simulink model "TSR_Scenario_001_cs"  (R2014b)
settings: Solver=ode5  SolverMode=SingleTasking  StartTime=0.0  StopTime=inf  FixedStep=1/100  RelTol=1e-3
PreLoadFcn:
  | mbxruntime.callbacks.PreLoadFcn(bdroot);
  | check_NUTS_defined;
  | 
  | assignin('base',['model_closed_' bdroot],false);
  | 
  | addpath('../includes_TSR/includes_TSR');
  | 
  | switch version('-release')
  | case {'2010a', '2010b', '2011a'}
  | addpath('../includes_TSR/ML2010b');
  | otherwise
  | addpath('../includes_TSR/ML2011b');
  | end
PostLoadFcn:
  | mbxruntime.callbacks.PostLoadFcn(bdroot);
InitFcn:
  | mbxruntime.callbacks.InitFcn(bdroot);
StartFcn:
  | mbxruntime.callbacks.StartFcn(bdroot);
StopFcn:
  | mbxruntime.callbacks.StopFcn(bdroot);
model workspace: external: MAT-File .\TSR_Scenario_001_cs_hws.mat (data not in the file)
undefined symbols (not defined in the file or in its folder): InitImageOutputDir, mbxruntime, OrientationPitch, OrientationRoll, PositionX, PositionY, PositionZ, tabledata, warningInitialVelocity, x0
undefined symbols (not defined in the file): SteeringColumn, SteeringWheel, TSR_Scenario_001_cs_0469e6db089af631, TSR_Scenario_001_cs_0511100212e7bc8e, TSR_Scenario_001_cs_0e7e9ae969427aac, TSR_Scenario_001_cs_1093386e49c2fe1f, TSR_Scenario_001_cs_112063adae8cf595, TSR_Scenario_001_cs_20f00d93cd5331c2, TSR_Scenario_001_cs_23e3512474fbfadc, TSR_Scenario_001_cs_366523e1554c6bf4, TSR_Scenario_001_cs_37bce4982c67337a, TSR_Scenario_001_cs_44e6164a5df50f45, TSR_Scenario_001_cs_4963ce12e7ff3247, TSR_Scenario_001_cs_4b3e01fa729ce73a, TSR_Scenario_001_cs_519c34727ce9f069, TSR_Scenario_001_cs_5b66ab60038399a1, TSR_Scenario_001_cs_5baa165dfa1afdcb, TSR_Scenario_001_cs_5f993ce39fa6372c, TSR_Scenario_001_cs_613fdf28e3ff7437, TSR_Scenario_001_cs_67b1406af835d622, TSR_Scenario_001_cs_6ad990c290286b94, TSR_Scenario_001_cs_6c412b69295984e1, TSR_Scenario_001_cs_6d4c0c06b1585ef3, TSR_Scenario_001_cs_6dd019d071bf1235, TSR_Scenario_001_cs_6e9f5883f1a78533, TSR_Scenario_001_cs_80f7223d9ac35404, TSR_Scenario_001_cs_8562b82d3c89ae57, TSR_Scenario_001_cs_8a3a0181ab0babfe, TSR_Scenario_001_cs_8c997348ce80deaf, TSR_Scenario_001_cs_925bd6a073d9fe25, TSR_Scenario_001_cs_961436216add6114, TSR_Scenario_001_cs_991a7959256b2c84, TSR_Scenario_001_cs_9a95ce2c2e753616, TSR_Scenario_001_cs_a98aa9562e8552a9, TSR_Scenario_001_cs_ab44ae81dbfb58cd, TSR_Scenario_001_cs_Actros_2541_2_Path_pathUniqueID, TSR_Scenario_001_cs_ae74836ade6bff5a, TSR_Scenario_001_cs_Audi_A8_1_Dynamics_Simple_initialPitch, TSR_Scenario_001_cs_Audi_A8_1_Dynamics_Simple_initialRoll, TSR_Scenario_001_cs_Audi_A8_1_Dynamics_Simple_initialX, TSR_Scenario_001_cs_Audi_A8_1_Dynamics_Simple_initialY, TSR_Scenario_001_cs_Audi_A8_1_Dynamics_Simple_initialYaw, TSR_Scenario_001_cs_Audi_A8_1_Dynamics_Simple_initialZ, TSR_Scenario_001_cs_Audi_A8_2_Path_pathUniqueID, TSR_Scenario_001_cs_Audi_A8_2_SpeedProfile_speedProfileUniqueID, TSR_Scenario_001_cs_b2eca4eb2fce349a, TSR_Scenario_001_cs_b7bac209c1f2549f, TSR_Scenario_001_cs_bf3dccb66d3255a4, TSR_Scenario_001_cs_bf4c1a5315e3f716, TSR_Scenario_001_cs_BMW_Z3_1_Path_pathUniqueID, TSR_Scenario_001_cs_BMW_Z3_1_SpeedProfile_speedProfileUniqueID, TSR_Scenario_001_cs_BMW_Z3_2_Path_pathUniqueID, TSR_Scenario_001_cs_BMW_Z3_2_SpeedProfile_speedProfileUniqueID, TSR_Scenario_001_cs_c4c8fc4bdece03a9, TSR_Scenario_001_cs_c964c86aa54ad92e, TSR_Scenario_001_cs_cb64d1ef85329755, TSR_Scenario_001_cs_Citroen_C3_1_Path_pathUniqueID, TSR_Scenario_001_cs_Citroen_C3_2_Path_pathUniqueID, TSR_Scenario_001_cs_Citroen_C3_3_Path_pathUniqueID, TSR_Scenario_001_cs_Citroen_C3_4_Path_pathUniqueID ... (+25)
libraries: simulink x21, PreScanSimulinkLibrary x17, simulink_extras x13
(part 7 of 30)

== system TSR_Scenario_001_cs/Toyota_Yaris_1 ==
  SELF_Toyota_Yaris_1 : Inport  Tag=inport/SelfPort  OutDataTypeStr=Bus: PRESCAN_SELFSENSORDATA  PortDimensions=1  SampleTime=1/100  BusOutputAsStruct=on
  ColorRegion_Exterior_color : Constant  Tag=VisuLightConst  Value=[255 255 224]
  Ground_{1..6} (6 alike) : Ground
  JointGroup_WheelDisplacement_V2R : Subsystem  Tag=mux/Wheels  mask(PreScan Velocity to Wheel Angle Block:){TimeStep=1/100, TireRadius=0.29}
      mask prompts: TimeStep "Auto Assigned: Time Step [s]"; TireRadius "Tire Radius [m]"
      settings: DeleteFcn=PreScanBlockDeleteFcn;
      mask Display: disp('Velocity\nto\nWheelAngle')
  Path : S-Function  Tag=Path  LoadFcn=load('PrescanMotionData.mat')  FunctionName=sfun_Path  Parameters=uniqueID, pathUniqueID, timestep  EnableBusSupport=off  mask(Path){uniqueID=1961, pathUniqueID=TSR_Scenario_001_cs_Toyota_Yaris_1_Path_pathUniqueID, timestep=1/100}
      mask prompts: uniqueID "Object Unique ID"; pathUniqueID "Path Unique ID"; timestep "MATLAB timestep:"
      mask help:
      | The path block outputs the position along a given trajectory.
      |
      | For more information, please click Help.
      mask Help: eval('openHelp(312)')
      mask Display: image(imread('Path.png'))
  SELF_Demux : Subsystem  Tag=demux/SelfPort  mask(PreScan Demux Block:){}
      mask help:
      | The SELF port shows (state) information of the actor itself. The outputs are position in the experiment's axis system and the GPS coordinates, and the object's absolute velocity and compass heading.
      |
      | For more information, please click Help.
      settings: DeleteFcn=PreScanBlockDeleteFcn;
      mask Help: eval('openHelp(462)')
      mask Display:
      | port_label('output',1,'x [m]')
      | port_label('output',2,'y [m]')
      | port_label('output',3,'z [m]','texmode','on')
      | port_label('output',4,'Rotx [deg]','texmode','on')
      | port_label('output',5,'Roty [deg]','texmode','on')
      | port_label('output',6,'Rotz [deg]','texmode','on')
      | port_label('output',7,'GPS lat [deg]','texmode','on')
      | port_label('output',8,'GPS long [deg]','texmode','on')
      | port_label('output',9,'GPS alt [m]','texmode','on')
      | port_label('output',10,'Velocity [m/s]')
      | port_label('output',11,'Heading [deg]')
      | port_label('output',12,'Yaw rate [deg/s]')
  STATE_Toyota_Yaris_1_rc : RateTransition  Tag=mux_rc/StatePort  OutPortSampleTimeOpt=Inherit
  SpeedProfile : S-Function  Tag=SpeedProfile  LoadFcn=load('PrescanMotionData.mat')  FunctionName=sfun_SpeedProfile  Parameters=speedProfileUniqueID, timestep  EnableBusSupport=off  mask(SpeedProfile){speedProfileUniqueID=TSR_Scenario_001_cs_dadaf9392218b438, timestep=1/100}
      mask prompts: speedProfileUniqueID "Speed Profile Unique ID"; timestep "MATLAB timestep:"
      mask help:
      | The speed profile block outputs the travelled distance, velocities and acceleration along a given path.
      |
      | For more information, please click Help.
      mask Help: eval('openHelp(312)')
      mask Display: image(imread('SpeedProfile.png'))
  Terminator_{1..11} (11 alike) : Terminator
  VISUColorRegion_Exterior_Mux : Subsystem  Tag=mux/MuxColorRegion  LoadFcn=load PrescanColorData  mask(PreScan User Interface: VisuTextureColor){}
      mask help:
      | The VisuTextureColor block provides a way to adapt the color of a vehicle.
      |
      | For more information, please click Help.
      settings: DeleteFcn=PreScanBlockDeleteFcn;
      mask Help: eval('openHelp(230)')
  WheelDisplacement_Mux : Subsystem  Tag=mux/JointGroup  mask(JointGroup){}
      mask help:
      | The JointGroup allows to control several Joints in one go, as defined for this particular model.
      | For more information, look in the PreScan manual in the section "Model Preparation Tool" -> "Joint Groups"
      |
      | For more information on the Joints simulink interface, press Help.
      mask Help: eval('openHelp(254)')
  STATE_Toyota_Yaris_1_bus : Outport  Tag=outport/StatePort  OutDataTypeStr=Bus: PRESCAN_STATEACTUATORDATA  PortDimensions=1  SampleTime=1/100
  WheelL0_Toyota_Yaris_1 : Outport  Tag=outport/JointActuator  Port=2  OutDataTypeStr=Bus: PRESCAN_POSE_DATA  SampleTime=1/100
  WheelL1_Toyota_Yaris_1 : Outport  Tag=outport/JointActuator  Port=3  OutDataTypeStr=Bus: PRESCAN_POSE_DATA  SampleTime=1/100
  WheelR0_Toyota_Yaris_1 : Outport  Tag=outport/JointActuator  Port=4  OutDataTypeStr=Bus: PRESCAN_POSE_DATA  SampleTime=1/100
  WheelR1_Toyota_Yaris_1 : Outport  Tag=outport/JointActuator  Port=5  OutDataTypeStr=Bus: PRESCAN_POSE_DATA  SampleTime=1/100
  VISUColorRegion_Exterior_Toyota_Yaris_1 : Outport  Tag=outport/ColorRegion  Port=6  OutDataTypeStr=Bus: PRESCAN_COLOR_DATA  PortDimensions=1  SampleTime=1/100
  wires:
  SELF_Demux/10(velocity [m/s]) -> JointGroup_WheelDisplacement_V2R/1(Velocity [m/s])
  STATE_Toyota_Yaris_1_rc/1 -> STATE_Toyota_Yaris_1_bus/1
  SpeedProfile/1 -> Path/1
  Path/1 -> STATE_Toyota_Yaris_1_rc/1
  SELF_Toyota_Yaris_1/1 -> SELF_Demux/1(SELF)
  WheelDisplacement_Mux/1(WheelL0_Toyota_Yaris_1) -> WheelL0_Toyota_Yaris_1/1
  WheelDisplacement_Mux/2(WheelL1_Toyota_Yaris_1) -> WheelL1_Toyota_Yaris_1/1
  WheelDisplacement_Mux/3(WheelR0_Toyota_Yaris_1) -> WheelR0_Toyota_Yaris_1/1
  WheelDisplacement_Mux/4(WheelR1_Toyota_Yaris_1) -> WheelR1_Toyota_Yaris_1/1
  JointGroup_WheelDisplacement_V2R/1(Rotation [rad]) -> WheelDisplacement_Mux/3(Rotation [rad])
  VISUColorRegion_Exterior_Mux/1(ColorRegion) -> VISUColorRegion_Exterior_Toyota_Yaris_1/1
  ColorRegion_Exterior_color/1 -> VISUColorRegion_Exterior_Mux/1(RGB [-,-,-])
  SELF_Demux/1(x [m]) -> Terminator_1/1
  SELF_Demux/2(y [m]) -> Terminator_2/1
  SELF_Demux/3(z [m]) -> Terminator_3/1
  SELF_Demux/4(rotx [deg]) -> Terminator_4/1
  SELF_Demux/5(roty [deg]) -> Terminator_5/1
  SELF_Demux/6(rotz [deg]) -> Terminator_6/1
  SELF_Demux/7(GPS lat [deg]) -> Terminator_7/1
  SELF_Demux/8(GPS long [deg]) -> Terminator_8/1
  SELF_Demux/9(GPS alt [m]) -> Terminator_9/1
  SELF_Demux/11(heading [deg]) -> Terminator_10/1
  SELF_Demux/12(yaw rate [deg/s]) -> Terminator_11/1
  Ground_1/1 -> WheelDisplacement_Mux/1(Steering Angle Front [rad])
  Ground_2/1 -> WheelDisplacement_Mux/2(Steering Angle Rear [rad])
  Ground_3/1 -> WheelDisplacement_Mux/4(zDisp FL [m])
  Ground_4/1 -> WheelDisplacement_Mux/5(zDisp FR [m])
  Ground_5/1 -> WheelDisplacement_Mux/6(zDisp RL [m])
  Ground_6/1 -> WheelDisplacement_Mux/7(zDisp RR [m])

== system TSR_Scenario_001_cs/VISUColorRegion_Exterior_Audi_A8_2 ==
  VISUColorRegion_Exterior_Audi_A8_2 : Inport  Tag=inport/ColorRegion  OutDataTypeStr=Bus: PRESCAN_COLOR_DATA  PortDimensions=1  SampleTime=1/100  BusOutputAsStruct=on
  Actuator : S-Function  FunctionName=sfun_ColorActuator  Parameters=mbxruntime.parameters.convert(UniqueID), mbxruntime.parameters.convert(WorldModelSubPath),tabledata, TimeStep  EnableBusSupport=off  mask(PreScan Sink Block: VisuTextureColor){UniqueID=1951, WorldModelSubPath=/recolorRegion:name=Exterior/targetColor, TimeStep=1/100}
      mask prompts: UniqueID "Parent Unique Identifier (auto-generated)"; WorldModelSubPath "WM SubPath(auto-generated)"; TimeStep "Simulink time step"
      mask help:
      | The VisuTextureColor block provides a way to adapt the color of a vehicle.
      |
      | For more information, please click Help.
      mask init:
      | [tabledata] = mbxruntime.parameters.table(UniqueID,WorldModelSubPath);
      mask Help: eval('openHelp(230)')
      mask Display: image(imread('TextureColor.png'))
  wires:
  VISUColorRegion_Exterior_Audi_A8_2/1 -> Actuator/1

== system TSR_Scenario_001_cs/VISUColorRegion_Exterior_BMW_Z3_1 ==
  VISUColorRegion_Exterior_BMW_Z3_1 : Inport  Tag=inport/ColorRegion  OutDataTypeStr=Bus: PRESCAN_COLOR_DATA  PortDimensions=1  SampleTime=1/100  BusOutputAsStruct=on
  Actuator : S-Function  FunctionName=sfun_ColorActuator  Parameters=mbxruntime.parameters.convert(UniqueID), mbxruntime.parameters.convert(WorldModelSubPath),tabledata, TimeStep  EnableBusSupport=off  mask(PreScan Sink Block: VisuTextureColor){UniqueID=1948, WorldModelSubPath=/recolorRegion:name=Exterior/targetColor, TimeStep=1/100}
      mask prompts: UniqueID "Parent Unique Identifier (auto-generated)"; WorldModelSubPath "WM SubPath(auto-generated)"; TimeStep "Simulink time step"
      mask help:
      | The VisuTextureColor block provides a way to adapt the color of a vehicle.
      |
      | For more information, please click Help.
      mask init:
      | [tabledata] = mbxruntime.parameters.table(UniqueID,WorldModelSubPath);
      mask Help: eval('openHelp(230)')
      mask Display: image(imread('TextureColor.png'))
  wires:
  VISUColorRegion_Exterior_BMW_Z3_1/1 -> Actuator/1

== system TSR_Scenario_001_cs/VISUColorRegion_Exterior_BMW_Z3_2 ==
  VISUColorRegion_Exterior_BMW_Z3_2 : Inport  Tag=inport/ColorRegion  OutDataTypeStr=Bus: PRESCAN_COLOR_DATA  PortDimensions=1  SampleTime=1/100  BusOutputAsStruct=on
  Actuator : S-Function  FunctionName=sfun_ColorActuator  Parameters=mbxruntime.parameters.convert(UniqueID), mbxruntime.parameters.convert(WorldModelSubPath),tabledata, TimeStep  EnableBusSupport=off  mask(PreScan Sink Block: VisuTextureColor){UniqueID=2024, WorldModelSubPath=/recolorRegion:name=Exterior/targetColor, TimeStep=1/100}
      mask prompts: UniqueID "Parent Unique Identifier (auto-generated)"; WorldModelSubPath "WM SubPath(auto-generated)"; TimeStep "Simulink time step"
      mask help:
      | The VisuTextureColor block provides a way to adapt the color of a vehicle.
      |
      | For more information, please click Help.
      mask init:
      | [tabledata] = mbxruntime.parameters.table(UniqueID,WorldModelSubPath);
      mask Help: eval('openHelp(230)')
      mask Display: image(imread('TextureColor.png'))
  wires:
  VISUColorRegion_Exterior_BMW_Z3_2/1 -> Actuator/1

== system TSR_Scenario_001_cs/VISUColorRegion_Exterior_Citroen_C3_1 ==
  VISUColorRegion_Exterior_Citroen_C3_1 : Inport  Tag=inport/ColorRegion  OutDataTypeStr=Bus: PRESCAN_COLOR_DATA  PortDimensions=1  SampleTime=1/100  BusOutputAsStruct=on
  Actuator : S-Function  FunctionName=sfun_ColorActuator  Parameters=mbxruntime.parameters.convert(UniqueID), mbxruntime.parameters.convert(WorldModelSubPath),tabledata, TimeStep  EnableBusSupport=off  mask(PreScan Sink Block: VisuTextureColor){UniqueID=1955, WorldModelSubPath=/recolorRegion:name=Exterior/targetColor, TimeStep=1/100}
      mask prompts: UniqueID "Parent Unique Identifier (auto-generated)"; WorldModelSubPath "WM SubPath(auto-generated)"; TimeStep "Simulink time step"
      mask help:
      | The VisuTextureColor block provides a way to adapt the color of a vehicle.
      |
      | For more information, please click Help.
      mask init:
      | [tabledata] = mbxruntime.parameters.table(UniqueID,WorldModelSubPath);
      mask Help: eval('openHelp(230)')
      mask Display: image(imread('TextureColor.png'))
  wires:
  VISUColorRegion_Exterior_Citroen_C3_1/1 -> Actuator/1

== system TSR_Scenario_001_cs/VISUColorRegion_Exterior_Citroen_C3_2 ==
  VISUColorRegion_Exterior_Citroen_C3_2 : Inport  Tag=inport/ColorRegion  OutDataTypeStr=Bus: PRESCAN_COLOR_DATA  PortDimensions=1  SampleTime=1/100  BusOutputAsStruct=on
  Actuator : S-Function  FunctionName=sfun_ColorActuator  Parameters=mbxruntime.parameters.convert(UniqueID), mbxruntime.parameters.convert(WorldModelSubPath),tabledata, TimeStep  EnableBusSupport=off  mask(PreScan Sink Block: VisuTextureColor){UniqueID=1958, WorldModelSubPath=/recolorRegion:name=Exterior/targetColor, TimeStep=1/100}
      mask prompts: UniqueID "Parent Unique Identifier (auto-generated)"; WorldModelSubPath "WM SubPath(auto-generated)"; TimeStep "Simulink time step"
      mask help:
      | The VisuTextureColor block provides a way to adapt the color of a vehicle.
      |
      | For more information, please click Help.
      mask init:
      | [tabledata] = mbxruntime.parameters.table(UniqueID,WorldModelSubPath);
      mask Help: eval('openHelp(230)')
      mask Display: image(imread('TextureColor.png'))
  wires:
  VISUColorRegion_Exterior_Citroen_C3_2/1 -> Actuator/1

== system TSR_Scenario_001_cs/VISUColorRegion_Exterior_Citroen_C3_3 ==
  VISUColorRegion_Exterior_Citroen_C3_3 : Inport  Tag=inport/ColorRegion  OutDataTypeStr=Bus: PRESCAN_COLOR_DATA  PortDimensions=1  SampleTime=1/100  BusOutputAsStruct=on
  Actuator : S-Function  FunctionName=sfun_ColorActuator  Parameters=mbxruntime.parameters.convert(UniqueID), mbxruntime.parameters.convert(WorldModelSubPath),tabledata, TimeStep  EnableBusSupport=off  mask(PreScan Sink Block: VisuTextureColor){UniqueID=1967, WorldModelSubPath=/recolorRegion:name=Exterior/targetColor, TimeStep=1/100}
      mask prompts: UniqueID "Parent Unique Identifier (auto-generated)"; WorldModelSubPath "WM SubPath(auto-generated)"; TimeStep "Simulink time step"
      mask help:
      | The VisuTextureColor block provides a way to adapt the color of a vehicle.
      |
      | For more information, please click Help.
      mask init:
      | [tabledata] = mbxruntime.parameters.table(UniqueID,WorldModelSubPath);
      mask Help: eval('openHelp(230)')
      mask Display: image(imread('TextureColor.png'))
  wires:
  VISUColorRegion_Exterior_Citroen_C3_3/1 -> Actuator/1

== system TSR_Scenario_001_cs/VISUColorRegion_Exterior_Citroen_C3_4 ==
  VISUColorRegion_Exterior_Citroen_C3_4 : Inport  Tag=inport/ColorRegion  OutDataTypeStr=Bus: PRESCAN_COLOR_DATA  PortDimensions=1  SampleTime=1/100  BusOutputAsStruct=on
  Actuator : S-Function  FunctionName=sfun_ColorActuator  Parameters=mbxruntime.parameters.convert(UniqueID), mbxruntime.parameters.convert(WorldModelSubPath),tabledata, TimeStep  EnableBusSupport=off  mask(PreScan Sink Block: VisuTextureColor){UniqueID=2027, WorldModelSubPath=/recolorRegion:name=Exterior/targetColor, TimeStep=1/100}
      mask prompts: UniqueID "Parent Unique Identifier (auto-generated)"; WorldModelSubPath "WM SubPath(auto-generated)"; TimeStep "Simulink time step"
      mask help:
      | The VisuTextureColor block provides a way to adapt the color of a vehicle.
      |
      | For more information, please click Help.
      mask init:
      | [tabledata] = mbxruntime.parameters.table(UniqueID,WorldModelSubPath);
      mask Help: eval('openHelp(230)')
      mask Display: image(imread('TextureColor.png'))
  wires:
  VISUColorRegion_Exterior_Citroen_C3_4/1 -> Actuator/1

== system TSR_Scenario_001_cs/VISUColorRegion_Exterior_Fiat_Bravo_1 ==
  VISUColorRegion_Exterior_Fiat_Bravo_1 : Inport  Tag=inport/ColorRegion  OutDataTypeStr=Bus: PRESCAN_COLOR_DATA  PortDimensions=1  SampleTime=1/100  BusOutputAsStruct=on
  Actuator : S-Function  FunctionName=sfun_ColorActuator  Parameters=mbxruntime.parameters.convert(UniqueID), mbxruntime.parameters.convert(WorldModelSubPath),tabledata, TimeStep  EnableBusSupport=off  mask(PreScan Sink Block: VisuTextureColor){UniqueID=1964, WorldModelSubPath=/recolorRegion:name=Exterior/targetColor, TimeStep=1/100}
      mask prompts: UniqueID "Parent Unique Identifier (auto-generated)"; WorldModelSubPath "WM SubPath(auto-generated)"; TimeStep "Simulink time step"
      mask help:
      | The VisuTextureColor block provides a way to adapt the color of a vehicle.
      |
      | For more information, please click Help.
      mask init:
      | [tabledata] = mbxruntime.parameters.table(UniqueID,WorldModelSubPath);
      mask Help: eval('openHelp(230)')
      mask Display: image(imread('TextureColor.png'))
  wires:
  VISUColorRegion_Exterior_Fiat_Bravo_1/1 -> Actuator/1

== system TSR_Scenario_001_cs/VISUColorRegion_Exterior_Ford_Fiesta_1 ==
  VISUColorRegion_Exterior_Ford_Fiesta_1 : Inport  Tag=inport/ColorRegion  OutDataTypeStr=Bus: PRESCAN_COLOR_DATA  PortDimensions=1  SampleTime=1/100  BusOutputAsStruct=on
  Actuator : S-Function  FunctionName=sfun_ColorActuator  Parameters=mbxruntime.parameters.convert(UniqueID), mbxruntime.parameters.convert(WorldModelSubPath),tabledata, TimeStep  EnableBusSupport=off  mask(PreScan Sink Block: VisuTextureColor){UniqueID=1934, WorldModelSubPath=/recolorRegion:name=Exterior/targetColor, TimeStep=1/100}
      mask prompts: UniqueID "Parent Unique Identifier (auto-generated)"; WorldModelSubPath "WM SubPath(auto-generated)"; TimeStep "Simulink time step"
      mask help:
      | The VisuTextureColor block provides a way to adapt the color of a vehicle.
      |
      | For more information, please click Help.
      mask init:
      | [tabledata] = mbxruntime.parameters.table(UniqueID,WorldModelSubPath);
      mask Help: eval('openHelp(230)')
      mask Display: image(imread('TextureColor.png'))
  wires:
  VISUColorRegion_Exterior_Ford_Fiesta_1/1 -> Actuator/1

== system TSR_Scenario_001_cs/VISUColorRegion_Exterior_Mazda_RX8_1 ==
  VISUColorRegion_Exterior_Mazda_RX8_1 : Inport  Tag=inport/ColorRegion  OutDataTypeStr=Bus: PRESCAN_COLOR_DATA  PortDimensions=1  SampleTime=1/100  BusOutputAsStruct=on
  Actuator : S-Function  FunctionName=sfun_ColorActuator  Parameters=mbxruntime.parameters.convert(UniqueID), mbxruntime.parameters.convert(WorldModelSubPath),tabledata, TimeStep  EnableBusSupport=off  mask(PreScan Sink Block: VisuTextureColor){UniqueID=1863, WorldModelSubPath=/recolorRegion:name=Exterior/targetColor, TimeStep=1/100}
      mask prompts: UniqueID "Parent Unique Identifier (auto-generated)"; WorldModelSubPath "WM SubPath(auto-generated)"; TimeStep "Simulink time step"
      mask help:
      | The VisuTextureColor block provides a way to adapt the color of a vehicle.
      |
      | For more information, please click Help.
      mask init:
      | [tabledata] = mbxruntime.parameters.table(UniqueID,WorldModelSubPath);
      mask Help: eval('openHelp(230)')
      mask Display: image(imread('TextureColor.png'))
  wires:
  VISUColorRegion_Exterior_Mazda_RX8_1/1 -> Actuator/1

== system TSR_Scenario_001_cs/VISUColorRegion_Exterior_Mazda_RX8_2 ==
  VISUColorRegion_Exterior_Mazda_RX8_2 : Inport  Tag=inport/ColorRegion  OutDataTypeStr=Bus: PRESCAN_COLOR_DATA  PortDimensions=1  SampleTime=1/100  BusOutputAsStruct=on
  Actuator : S-Function  FunctionName=sfun_ColorActuator  Parameters=mbxruntime.parameters.convert(UniqueID), mbxruntime.parameters.convert(WorldModelSubPath),tabledata, TimeStep  EnableBusSupport=off  mask(PreScan Sink Block: VisuTextureColor){UniqueID=1929, WorldModelSubPath=/recolorRegion:name=Exterior/targetColor, TimeStep=1/100}
      mask prompts: UniqueID "Parent Unique Identifier (auto-generated)"; WorldModelSubPath "WM SubPath(auto-generated)"; TimeStep "Simulink time step"
      mask help:
      | The VisuTextureColor block provides a way to adapt the color of a vehicle.
      |
      | For more information, please click Help.
      mask init:
      | [tabledata] = mbxruntime.parameters.table(UniqueID,WorldModelSubPath);
      mask Help: eval('openHelp(230)')
      mask Display: image(imread('TextureColor.png'))
  wires:
  VISUColorRegion_Exterior_Mazda_RX8_2/1 -> Actuator/1

== system TSR_Scenario_001_cs/VISUColorRegion_Exterior_Mazda_RX8_3 ==
  VISUColorRegion_Exterior_Mazda_RX8_3 : Inport  Tag=inport/ColorRegion  OutDataTypeStr=Bus: PRESCAN_COLOR_DATA  PortDimensions=1  SampleTime=1/100  BusOutputAsStruct=on
  Actuator : S-Function  FunctionName=sfun_ColorActuator  Parameters=mbxruntime.parameters.convert(UniqueID), mbxruntime.parameters.convert(WorldModelSubPath),tabledata, TimeStep  EnableBusSupport=off  mask(PreScan Sink Block: VisuTextureColor){UniqueID=1973, WorldModelSubPath=/recolorRegion:name=Exterior/targetColor, TimeStep=1/100}
      mask prompts: UniqueID "Parent Unique Identifier (auto-generated)"; WorldModelSubPath "WM SubPath(auto-generated)"; TimeStep "Simulink time step"
      mask help:
      | The VisuTextureColor block provides a way to adapt the color of a vehicle.
      |
      | For more information, please click Help.
      mask init:
      | [tabledata] = mbxruntime.parameters.table(UniqueID,WorldModelSubPath);
      mask Help: eval('openHelp(230)')
      mask Display: image(imread('TextureColor.png'))
  wires:
  VISUColorRegion_Exterior_Mazda_RX8_3/1 -> Actuator/1

== system TSR_Scenario_001_cs/VISUColorRegion_Exterior_Nissan_Cabstar_1 ==
  VISUColorRegion_Exterior_Nissan_Cabstar_1 : Inport  Tag=inport/ColorRegion  OutDataTypeStr=Bus: PRESCAN_COLOR_DATA  PortDimensions=1  SampleTime=1/100  BusOutputAsStruct=on
  Actuator : S-Function  FunctionName=sfun_ColorActuator  Parameters=mbxruntime.parameters.convert(UniqueID), mbxruntime.parameters.convert(WorldModelSubPath),tabledata, TimeStep  EnableBusSupport=off  mask(PreScan Sink Block: VisuTextureColor){UniqueID=1579, WorldModelSubPath=/recolorRegion:name=Exterior/targetColor, TimeStep=1/100}
      mask prompts: UniqueID "Parent Unique Identifier (auto-generated)"; WorldModelSubPath "WM SubPath(auto-generated)"; TimeStep "Simulink time step"
      mask help:
      | The VisuTextureColor block provides a way to adapt the color of a vehicle.
      |
      | For more information, please click Help.
      mask init:
      | [tabledata] = mbxruntime.parameters.table(UniqueID,WorldModelSubPath);
      mask Help: eval('openHelp(230)')
      mask Display: image(imread('TextureColor.png'))
  wires:
  VISUColorRegion_Exterior_Nissan_Cabstar_1/1 -> Actuator/1

== system TSR_Scenario_001_cs/VISUColorRegion_Exterior_Toyota_Previa_1 ==
  VISUColorRegion_Exterior_Toyota_Previa_1 : Inport  Tag=inport/ColorRegion  OutDataTypeStr=Bus: PRESCAN_COLOR_DATA  PortDimensions=1  SampleTime=1/100  BusOutputAsStruct=on
  Actuator : S-Function  FunctionName=sfun_ColorActuator  Parameters=mbxruntime.parameters.convert(UniqueID), mbxruntime.parameters.convert(WorldModelSubPath),tabledata, TimeStep  EnableBusSupport=off  mask(PreScan Sink Block: VisuTextureColor){UniqueID=1688, WorldModelSubPath=/recolorRegion:name=Exterior/targetColor, TimeStep=1/100}
      mask prompts: UniqueID "Parent Unique Identifier (auto-generated)"; WorldModelSubPath "WM SubPath(auto-generated)"; TimeStep "Simulink time step"
      mask help:
      | The VisuTextureColor block provides a way to adapt the color of a vehicle.
      |
      | For more information, please click Help.
      mask init:
      | [tabledata] = mbxruntime.parameters.table(UniqueID,WorldModelSubPath);
      mask Help: eval('openHelp(230)')
      mask Display: image(imread('TextureColor.png'))
  wires:
  VISUColorRegion_Exterior_Toyota_Previa_1/1 -> Actuator/1

== system TSR_Scenario_001_cs/VISUColorRegion_Exterior_Toyota_Previa_2 ==
  VISUColorRegion_Exterior_Toyota_Previa_2 : Inport  Tag=inport/ColorRegion  OutDataTypeStr=Bus: PRESCAN_COLOR_DATA  PortDimensions=1  SampleTime=1/100  BusOutputAsStruct=on
  Actuator : S-Function  FunctionName=sfun_ColorActuator  Parameters=mbxruntime.parameters.convert(UniqueID), mbxruntime.parameters.convert(WorldModelSubPath),tabledata, TimeStep  EnableBusSupport=off  mask(PreScan Sink Block: VisuTextureColor){UniqueID=1970, WorldModelSubPath=/recolorRegion:name=Exterior/targetColor, TimeStep=1/100}
      mask prompts: UniqueID "Parent Unique Identifier (auto-generated)"; WorldModelSubPath "WM SubPath(auto-generated)"; TimeStep "Simulink time step"
      mask help:
      | The VisuTextureColor block provides a way to adapt the color of a vehicle.
      |
      | For more information, please click Help.
      mask init:
      | [tabledata] = mbxruntime.parameters.table(UniqueID,WorldModelSubPath);
      mask Help: eval('openHelp(230)')
      mask Display: image(imread('TextureColor.png'))
  wires:
  VISUColorRegion_Exterior_Toyota_Previa_2/1 -> Actuator/1

== system TSR_Scenario_001_cs/VISUColorRegion_Exterior_Toyota_Yaris_1 ==
  VISUColorRegion_Exterior_Toyota_Yaris_1 : Inport  Tag=inport/ColorRegion  OutDataTypeStr=Bus: PRESCAN_COLOR_DATA  PortDimensions=1  SampleTime=1/100  BusOutputAsStruct=on
  Actuator : S-Function  FunctionName=sfun_ColorActuator  Parameters=mbxruntime.parameters.convert(UniqueID), mbxruntime.parameters.convert(WorldModelSubPath),tabledata, TimeStep  EnableBusSupport=off  mask(PreScan Sink Block: VisuTextureColor){UniqueID=1961, WorldModelSubPath=/recolorRegion:name=Exterior/targetColor, TimeStep=1/100}
      mask prompts: UniqueID "Parent Unique Identifier (auto-generated)"; WorldModelSubPath "WM SubPath(auto-generated)"; TimeStep "Simulink time step"
      mask help:
      | The VisuTextureColor block provides a way to adapt the color of a vehicle.
      |
      | For more information, please click Help.
      mask init:
      | [tabledata] = mbxruntime.parameters.table(UniqueID,WorldModelSubPath);
      mask Help: eval('openHelp(230)')
      mask Display: image(imread('TextureColor.png'))
  wires:
  VISUColorRegion_Exterior_Toyota_Yaris_1/1 -> Actuator/1

== system TSR_Scenario_001_cs/VISUMatrixSignLights_HighwayOverhang_1 ==
  VISUMatrixSignLights_HighwayOverhang_1 : Inport  Tag=inport/VisuMatrixSignLights  SampleTime=1/100  BusOutputAsStruct=on
  Actuator : Subsystem  mask(PreScan Sink Block: VisuMatrixSignLights){UniqueID=1876, ColorsObjectQuery=, Colors=[]}
      mask prompts: UniqueID "Parent Unique Identifier"; ColorsObjectQuery "Query for Color Object"; Colors "Matrix of colors"
      mask help:
      | The VisuMatrixSignLights block provides a way to switch the lights on the matrix sign board on or off
      |
      | For more information, please click Help.
      mask Help: eval('openHelp(732)')
      mask Display: image(imread('RearLight.png'))
  wires:
  VISUMatrixSignLights_HighwayOverhang_1/1 -> Actuator/1(VISUMatrixSignLights_HighwayOverhang_1)

== system TSR_Scenario_001_cs/VISUMatrixSignLights_HighwayOverhang_2 ==
  VISUMatrixSignLights_HighwayOverhang_2 : Inport  Tag=inport/VisuMatrixSignLights  SampleTime=1/100  BusOutputAsStruct=on
  Actuator : Subsystem  mask(PreScan Sink Block: VisuMatrixSignLights){UniqueID=1877, ColorsObjectQuery=, Colors=[]}
      mask prompts: UniqueID "Parent Unique Identifier"; ColorsObjectQuery "Query for Color Object"; Colors "Matrix of colors"
      mask help:
      | The VisuMatrixSignLights block provides a way to switch the lights on the matrix sign board on or off
      |
      | For more information, please click Help.
      mask Help: eval('openHelp(732)')
      mask Display: image(imread('RearLight.png'))
  wires:
  VISUMatrixSignLights_HighwayOverhang_2/1 -> Actuator/1(VISUMatrixSignLights_HighwayOverhang_2)

== system TSR_Scenario_001_cs/VISUMatrixSignLights_HighwayOverhang_3 ==
  VISUMatrixSignLights_HighwayOverhang_3 : Inport  Tag=inport/VisuMatrixSignLights  SampleTime=1/100  BusOutputAsStruct=on
  Actuator : Subsystem  mask(PreScan Sink Block: VisuMatrixSignLights){UniqueID=1890, ColorsObjectQuery=, Colors=[]}
      mask prompts: UniqueID "Parent Unique Identifier"; ColorsObjectQuery "Query for Color Object"; Colors "Matrix of colors"
      mask help:
      | The VisuMatrixSignLights block provides a way to switch the lights on the matrix sign board on or off
      |
      | For more information, please click Help.
      mask Help: eval('openHelp(732)')
      mask Display: image(imread('RearLight.png'))
  wires:
  VISUMatrixSignLights_HighwayOverhang_3/1 -> Actuator/1(VISUMatrixSignLights_HighwayOverhang_3)

== system TSR_Scenario_001_cs/VISUMatrixSignLights_HighwayOverhang_4 ==
  VISUMatrixSignLights_HighwayOverhang_4 : Inport  Tag=inport/VisuMatrixSignLights  SampleTime=1/100  BusOutputAsStruct=on
  Actuator : Subsystem  mask(PreScan Sink Block: VisuMatrixSignLights){UniqueID=1898, ColorsObjectQuery=, Colors=[]}
      mask prompts: UniqueID "Parent Unique Identifier"; ColorsObjectQuery "Query for Color Object"; Colors "Matrix of colors"
      mask help:
      | The VisuMatrixSignLights block provides a way to switch the lights on the matrix sign board on or off
      |
      | For more information, please click Help.
      mask Help: eval('openHelp(732)')
      mask Display: image(imread('RearLight.png'))
  wires:
  VISUMatrixSignLights_HighwayOverhang_4/1 -> Actuator/1(VISUMatrixSignLights_HighwayOverhang_4)

== system TSR_Scenario_001_cs/VISUMatrixSignLights_HighwayOverhang_5 ==
  VISUMatrixSignLights_HighwayOverhang_5 : Inport  Tag=inport/VisuMatrixSignLights  SampleTime=1/100  BusOutputAsStruct=on
  Actuator : Subsystem  mask(PreScan Sink Block: VisuMatrixSignLights){UniqueID=1909, ColorsObjectQuery=, Colors=[]}
      mask prompts: UniqueID "Parent Unique Identifier"; ColorsObjectQuery "Query for Color Object"; Colors "Matrix of colors"
      mask help:
      | The VisuMatrixSignLights block provides a way to switch the lights on the matrix sign board on or off
      |
      | For more information, please click Help.
      mask Help: eval('openHelp(732)')
      mask Display: image(imread('RearLight.png'))
  wires:
  VISUMatrixSignLights_HighwayOverhang_5/1 -> Actuator/1(VISUMatrixSignLights_HighwayOverhang_5)

== system TSR_Scenario_001_cs/VISUMatrixSignLights_HighwayOverhang_6 ==
  VISUMatrixSignLights_HighwayOverhang_6 : Inport  Tag=inport/VisuMatrixSignLights  SampleTime=1/100  BusOutputAsStruct=on
  Actuator : Subsystem  mask(PreScan Sink Block: VisuMatrixSignLights){UniqueID=1914, ColorsObjectQuery=, Colors=[]}
      mask prompts: UniqueID "Parent Unique Identifier"; ColorsObjectQuery "Query for Color Object"; Colors "Matrix of colors"
      mask help:
      | The VisuMatrixSignLights block provides a way to switch the lights on the matrix sign board on or off
      |
      | For more information, please click Help.
      mask Help: eval('openHelp(732)')
      mask Display: image(imread('RearLight.png'))
  wires:
  VISUMatrixSignLights_HighwayOverhang_6/1 -> Actuator/1(VISUMatrixSignLights_HighwayOverhang_6)

== system TSR_Scenario_001_cs/VISUMatrixSign_HighwayOverhang_1 ==
  VISUMatrixSign_HighwayOverhang_1 : Inport  Tag=inport/VisuMatrixSign  SampleTime=1/100  BusOutputAsStruct=on
  Actuator : Subsystem  mask(PreScan Sink Block: VisuMatrixSign){UniqueID=1876, ResourceList={'3' 'InformationSign\MatrixSign_Empty.png' '4' 'InformationSign\MatrixSign_End.png' '5' 'InformationSign\MatrixSign_GreenArrow.png' '6' 'InformationSign\MatrixSign_RedCross.png' '7' 'InformationSign\MatrixSign_Speed_50.png' '8' 'InformationSign\MatrixSign_Speed_70.png' '9' 'InformationSign\MatrixSign_Speed_90.png' '10' 'InformationSign\MatrixSign_Speed_120.png' '11' 'InformationSign\MatrixSign_Speed_130.png' '12' 'InformationSign\information.png' '13' 'InformationSign\Empty.jpg' }, PivotName=}
      mask prompts: UniqueID "Parent Unique Identifier (auto-generated)"; ResourceList "Resource List (auto-generated)"; PivotName "Name of pivot (auto-generated)"
      mask help:
      | The VisuMatrixSign block provides a way to adapt the texture of the plates connected to an overhang, based on Resource IDs of the texture files.
      |
      | For more information, please click Help.
      mask Help: eval('openHelp(733)')
      mask Display: image(imread('HighwaySpeedMatrix.png'))
  wires:
  VISUMatrixSign_HighwayOverhang_1/1 -> Actuator/1(VISUMatrixSign_HighwayOverhang_1)

== system TSR_Scenario_001_cs/VISUMatrixSign_HighwayOverhang_2 ==
  VISUMatrixSign_HighwayOverhang_2 : Inport  Tag=inport/VisuMatrixSign  SampleTime=1/100  BusOutputAsStruct=on
  Actuator : Subsystem  mask(PreScan Sink Block: VisuMatrixSign){UniqueID=1877, ResourceList={'3' 'InformationSign\MatrixSign_Empty.png' '4' 'InformationSign\MatrixSign_End.png' '5' 'InformationSign\MatrixSign_GreenArrow.png' '6' 'InformationSign\MatrixSign_RedCross.png' '7' 'InformationSign\MatrixSign_Speed_50.png' '8' 'InformationSign\MatrixSign_Speed_70.png' '9' 'InformationSign\MatrixSign_Speed_90.png' '10' 'InformationSign\MatrixSign_Speed_120.png' '11' 'InformationSign\MatrixSign_Speed_130.png' '12' 'InformationSign\information.png' '13' 'InformationSign\Empty.jpg' }, PivotName=}
      mask prompts: UniqueID "Parent Unique Identifier (auto-generated)"; ResourceList "Resource List (auto-generated)"; PivotName "Name of pivot (auto-generated)"
      mask help:
      | The VisuMatrixSign block provides a way to adapt the texture of the plates connected to an overhang, based on Resource IDs of the texture files.
      |
      | For more information, please click Help.
      mask Help: eval('openHelp(733)')
      mask Display: image(imread('HighwaySpeedMatrix.png'))
  wires:
  VISUMatrixSign_HighwayOverhang_2/1 -> Actuator/1(VISUMatrixSign_HighwayOverhang_2)

== system TSR_Scenario_001_cs/VISUMatrixSign_HighwayOverhang_3 ==
  VISUMatrixSign_HighwayOverhang_3 : Inport  Tag=inport/VisuMatrixSign  SampleTime=1/100  BusOutputAsStruct=on
  Actuator : Subsystem  mask(PreScan Sink Block: VisuMatrixSign){UniqueID=1890, ResourceList={'3' 'InformationSign\MatrixSign_Empty.png' '4' 'InformationSign\MatrixSign_End.png' '5' 'InformationSign\MatrixSign_GreenArrow.png' '6' 'InformationSign\MatrixSign_RedCross.png' '7' 'InformationSign\MatrixSign_Speed_50.png' '8' 'InformationSign\MatrixSign_Speed_70.png' '9' 'InformationSign\MatrixSign_Speed_90.png' '10' 'InformationSign\MatrixSign_Speed_120.png' '11' 'InformationSign\MatrixSign_Speed_130.png' '12' 'InformationSign\information.png' '13' 'InformationSign\Empty.jpg' }, PivotName=}
      mask prompts: UniqueID "Parent Unique Identifier (auto-generated)"; ResourceList "Resource List (auto-generated)"; PivotName "Name of pivot (auto-generated)"
      mask help:
      | The VisuMatrixSign block provides a way to adapt the texture of the plates connected to an overhang, based on Resource IDs of the texture files.
      |
      | For more information, please click Help.
      mask Help: eval('openHelp(733)')
      mask Display: image(imread('HighwaySpeedMatrix.png'))
  wires:
  VISUMatrixSign_HighwayOverhang_3/1 -> Actuator/1(VISUMatrixSign_HighwayOverhang_3)

== system TSR_Scenario_001_cs/VISUMatrixSign_HighwayOverhang_4 ==
  VISUMatrixSign_HighwayOverhang_4 : Inport  Tag=inport/VisuMatrixSign  SampleTime=1/100  BusOutputAsStruct=on
  Actuator : Subsystem  mask(PreScan Sink Block: VisuMatrixSign){UniqueID=1898, ResourceList={'3' 'InformationSign\MatrixSign_Empty.png' '4' 'InformationSign\MatrixSign_End.png' '5' 'InformationSign\MatrixSign_GreenArrow.png' '6' 'InformationSign\MatrixSign_RedCross.png' '7' 'InformationSign\MatrixSign_Speed_50.png' '8' 'InformationSign\MatrixSign_Speed_70.png' '9' 'InformationSign\MatrixSign_Speed_90.png' '10' 'InformationSign\MatrixSign_Speed_120.png' '11' 'InformationSign\MatrixSign_Speed_130.png' '12' 'InformationSign\information.png' '13' 'InformationSign\Empty.jpg' }, PivotName=}
      mask prompts: UniqueID "Parent Unique Identifier (auto-generated)"; ResourceList "Resource List (auto-generated)"; PivotName "Name of pivot (auto-generated)"
      mask help:
      | The VisuMatrixSign block provides a way to adapt the texture of the plates connected to an overhang, based on Resource IDs of the texture files.
      |
      | For more information, please click Help.
      mask Help: eval('openHelp(733)')
      mask Display: image(imread('HighwaySpeedMatrix.png'))
  wires:
  VISUMatrixSign_HighwayOverhang_4/1 -> Actuator/1(VISUMatrixSign_HighwayOverhang_4)

== system TSR_Scenario_001_cs/VISUMatrixSign_HighwayOverhang_5 ==
  VISUMatrixSign_HighwayOverhang_5 : Inport  Tag=inport/VisuMatrixSign  SampleTime=1/100  BusOutputAsStruct=on
  Actuator : Subsystem  mask(PreScan Sink Block: VisuMatrixSign){UniqueID=1909, ResourceList={'3' 'InformationSign\MatrixSign_Empty.png' '4' 'InformationSign\MatrixSign_End.png' '5' 'InformationSign\MatrixSign_GreenArrow.png' '6' 'InformationSign\MatrixSign_RedCross.png' '7' 'InformationSign\MatrixSign_Speed_50.png' '8' 'InformationSign\MatrixSign_Speed_70.png' '9' 'InformationSign\MatrixSign_Speed_90.png' '10' 'InformationSign\MatrixSign_Speed_120.png' '11' 'InformationSign\MatrixSign_Speed_130.png' '12' 'InformationSign\information.png' '13' 'InformationSign\Empty.jpg' }, PivotName=}
      mask prompts: UniqueID "Parent Unique Identifier (auto-generated)"; ResourceList "Resource List (auto-generated)"; PivotName "Name of pivot (auto-generated)"
      mask help:
      | The VisuMatrixSign block provides a way to adapt the texture of the plates connected to an overhang, based on Resource IDs of the texture files.
      |
      | For more information, please click Help.
      mask Help: eval('openHelp(733)')
      mask Display: image(imread('HighwaySpeedMatrix.png'))
  wires:
  VISUMatrixSign_HighwayOverhang_5/1 -> Actuator/1(VISUMatrixSign_HighwayOverhang_5)

== system TSR_Scenario_001_cs/VISUMatrixSign_HighwayOverhang_6 ==
  VISUMatrixSign_HighwayOverhang_6 : Inport  Tag=inport/VisuMatrixSign  SampleTime=1/100  BusOutputAsStruct=on
  Actuator : Subsystem  mask(PreScan Sink Block: VisuMatrixSign){UniqueID=1914, ResourceList={'3' 'InformationSign\MatrixSign_Empty.png' '4' 'InformationSign\MatrixSign_End.png' '5' 'InformationSign\MatrixSign_GreenArrow.png' '6' 'InformationSign\MatrixSign_RedCross.png' '7' 'InformationSign\MatrixSign_Speed_50.png' '8' 'InformationSign\MatrixSign_Speed_70.png' '9' 'InformationSign\MatrixSign_Speed_90.png' '10' 'InformationSign\MatrixSign_Speed_120.png' '11' 'InformationSign\MatrixSign_Speed_130.png' '12' 'InformationSign\information.png' '13' 'InformationSign\Empty.jpg' }, PivotName=}
      mask prompts: UniqueID "Parent Unique Identifier (auto-generated)"; ResourceList "Resource List (auto-generated)"; PivotName "Name of pivot (auto-generated)"
      mask help:
      | The VisuMatrixSign block provides a way to adapt the texture of the plates connected to an overhang, based on Resource IDs of the texture files.
      |
      | For more information, please click Help.
      mask Help: eval('openHelp(733)')
      mask Display: image(imread('HighwaySpeedMatrix.png'))
  wires:
  VISUMatrixSign_HighwayOverhang_6/1 -> Actuator/1(VISUMatrixSign_HighwayOverhang_6)

== system TSR_Scenario_001_cs/VISUMatrixSign_HighwayOverhang_7 ==
  VISUMatrixSign_HighwayOverhang_7 : Inport  Tag=inport/VisuMatrixSign  SampleTime=1/100  BusOutputAsStruct=on
  Actuator : Subsystem  mask(PreScan Sink Block: VisuMatrixSign){UniqueID=2612, ResourceList={'3' 'InformationSign\MatrixSign_Empty.png' '4' 'InformationSign\MatrixSign_End.png' '5' 'InformationSign\MatrixSign_GreenArrow.png' '6' 'InformationSign\MatrixSign_RedCross.png' '7' 'InformationSign\MatrixSign_Speed_50.png' '8' 'InformationSign\MatrixSign_Speed_70.png' '9' 'InformationSign\MatrixSign_Speed_90.png' '10' 'InformationSign\MatrixSign_Speed_120.png' '11' 'InformationSign\MatrixSign_Speed_130.png' '12' 'InformationSign\information.png' '13' 'InformationSign\Empty.jpg' }, PivotName=}
      mask prompts: UniqueID "Parent Unique Identifier (auto-generated)"; ResourceList "Resource List (auto-generated)"; PivotName "Name of pivot (auto-generated)"
      mask help:
      | The VisuMatrixSign block provides a way to adapt the texture of the plates connected to an overhang, based on Resource IDs of the texture files.
      |
      | For more information, please click Help.
      mask Help: eval('openHelp(733)')
      mask Display: image(imread('HighwaySpeedMatrix.png'))
  wires:
  VISUMatrixSign_HighwayOverhang_7/1 -> Actuator/1(VISUMatrixSign_HighwayOverhang_7)

== system TSR_Scenario_001_cs/WheelL0_Actros_2541_2 ==
  WheelL0_Actros_2541_2 : Inport  Tag=inport/JointActuator  OutDataTypeStr=Bus: PRESCAN_POSE_DATA  SampleTime=1/100  BusOutputAsStruct=on
  Actuator : Subsystem  Tag=VisuJoint  mask(PreScan Sink Block: VisuJoint){UniqueID=2575, Translate_ObjectID3D=Actros_2541_2.WheelL0, Rotate_ObjectID3D=Actros_2541_2.WheelL0, TimeStep=1/100, DisplayName=[]}
      mask prompts: UniqueID "Parent Unique ID"; Translate_ObjectID3D "Translate Object Name"; Rotate_ObjectID3D "Rotate Object Name"; TimeStep "Simulation Step"; DisplayName "Display Name"
      mask help:
      | The VisuJoint block provides a way to adapt the location and orientation of a part of an object.
      |
      | For more information, please click Help.
      settings: DeleteFcn=PreScanBlockDeleteFcn;
      mask Help: eval('openHelp(223)')
      mask Display: image(imread('Joint.png'))
  wires:
  WheelL0_Actros_2541_2/1 -> Actuator/1(Joint)

== system TSR_Scenario_001_cs/WheelL0_Audi_A8_1 ==
  WheelL0_Audi_A8_1 : Inport  Tag=inport/JointActuator  OutDataTypeStr=Bus: PRESCAN_POSE_DATA  SampleTime=1/100  BusOutputAsStruct=on
  Actuator : Subsystem  Tag=VisuJoint  mask(PreScan Sink Block: VisuJoint){UniqueID=253, Translate_ObjectID3D=Audi_A8_1.WheelL0, Rotate_ObjectID3D=Audi_A8_1.WheelL0, TimeStep=1/100, DisplayName=[]}
      mask prompts: UniqueID "Parent Unique ID"; Translate_ObjectID3D "Translate Object Name"; Rotate_ObjectID3D "Rotate Object Name"; TimeStep "Simulation Step"; DisplayName "Display Name"
      mask help:
      | The VisuJoint block provides a way to adapt the location and orientation of a part of an object.
      |
      | For more information, please click Help.
      settings: DeleteFcn=PreScanBlockDeleteFcn;
      mask Help: eval('openHelp(223)')
      mask Display: image(imread('Joint.png'))
  wires:
  WheelL0_Audi_A8_1/1 -> Actuator/1(Joint)

== system TSR_Scenario_001_cs/WheelL0_Audi_A8_2 ==
  WheelL0_Audi_A8_2 : Inport  Tag=inport/JointActuator  OutDataTypeStr=Bus: PRESCAN_POSE_DATA  SampleTime=1/100  BusOutputAsStruct=on
  Actuator : Subsystem  Tag=VisuJoint  mask(PreScan Sink Block: VisuJoint){UniqueID=1951, Translate_ObjectID3D=Audi_A8_2.WheelL0, Rotate_ObjectID3D=Audi_A8_2.WheelL0, TimeStep=1/100, DisplayName=[]}
      mask prompts: UniqueID "Parent Unique ID"; Translate_ObjectID3D "Translate Object Name"; Rotate_ObjectID3D "Rotate Object Name"; TimeStep "Simulation Step"; DisplayName "Display Name"
      mask help:
      | The VisuJoint block provides a way to adapt the location and orientation of a part of an object.
      |
      | For more information, please click Help.
      settings: DeleteFcn=PreScanBlockDeleteFcn;
      mask Help: eval('openHelp(223)')
      mask Display: image(imread('Joint.png'))
  wires:
  WheelL0_Audi_A8_2/1 -> Actuator/1(Joint)

== system TSR_Scenario_001_cs/WheelL0_BMW_Z3_1 ==
  WheelL0_BMW_Z3_1 : Inport  Tag=inport/JointActuator  OutDataTypeStr=Bus: PRESCAN_POSE_DATA  SampleTime=1/100  BusOutputAsStruct=on
  Actuator : Subsystem  Tag=VisuJoint  mask(PreScan Sink Block: VisuJoint){UniqueID=1948, Translate_ObjectID3D=BMW_Z3_1.WheelL0, Rotate_ObjectID3D=BMW_Z3_1.WheelL0, TimeStep=1/100, DisplayName=[]}
      mask prompts: UniqueID "Parent Unique ID"; Translate_ObjectID3D "Translate Object Name"; Rotate_ObjectID3D "Rotate Object Name"; TimeStep "Simulation Step"; DisplayName "Display Name"
      mask help:
      | The VisuJoint block provides a way to adapt the location and orientation of a part of an object.
      |
      | For more information, please click Help.
      settings: DeleteFcn=PreScanBlockDeleteFcn;
      mask Help: eval('openHelp(223)')
      mask Display: image(imread('Joint.png'))
  wires:
  WheelL0_BMW_Z3_1/1 -> Actuator/1(Joint)

== system TSR_Scenario_001_cs/WheelL0_BMW_Z3_2 ==
  WheelL0_BMW_Z3_2 : Inport  Tag=inport/JointActuator  OutDataTypeStr=Bus: PRESCAN_POSE_DATA  SampleTime=1/100  BusOutputAsStruct=on
  Actuator : Subsystem  Tag=VisuJoint  mask(PreScan Sink Block: VisuJoint){UniqueID=2024, Translate_ObjectID3D=BMW_Z3_2.WheelL0, Rotate_ObjectID3D=BMW_Z3_2.WheelL0, TimeStep=1/100, DisplayName=[]}
      mask prompts: UniqueID "Parent Unique ID"; Translate_ObjectID3D "Translate Object Name"; Rotate_ObjectID3D "Rotate Object Name"; TimeStep "Simulation Step"; DisplayName "Display Name"
      mask help:
      | The VisuJoint block provides a way to adapt the location and orientation of a part of an object.
      |
      | For more information, please click Help.
      settings: DeleteFcn=PreScanBlockDeleteFcn;
      mask Help: eval('openHelp(223)')
      mask Display: image(imread('Joint.png'))
  wires:
  WheelL0_BMW_Z3_2/1 -> Actuator/1(Joint)

== system TSR_Scenario_001_cs/WheelL0_Citroen_C3_1 ==
  WheelL0_Citroen_C3_1 : Inport  Tag=inport/JointActuator  OutDataTypeStr=Bus: PRESCAN_POSE_DATA  SampleTime=1/100  BusOutputAsStruct=on
  Actuator : Subsystem  Tag=VisuJoint  mask(PreScan Sink Block: VisuJoint){UniqueID=1955, Translate_ObjectID3D=Citroen_C3_1.WheelL0, Rotate_ObjectID3D=Citroen_C3_1.WheelL0, TimeStep=1/100, DisplayName=[]}
      mask prompts: UniqueID "Parent Unique ID"; Translate_ObjectID3D "Translate Object Name"; Rotate_ObjectID3D "Rotate Object Name"; TimeStep "Simulation Step"; DisplayName "Display Name"
      mask help:
      | The VisuJoint block provides a way to adapt the location and orientation of a part of an object.
      |
      | For more information, please click Help.
      settings: DeleteFcn=PreScanBlockDeleteFcn;
      mask Help: eval('openHelp(223)')
      mask Display: image(imread('Joint.png'))
  wires:
  WheelL0_Citroen_C3_1/1 -> Actuator/1(Joint)

== system TSR_Scenario_001_cs/WheelL0_Citroen_C3_2 ==
  WheelL0_Citroen_C3_2 : Inport  Tag=inport/JointActuator  OutDataTypeStr=Bus: PRESCAN_POSE_DATA  SampleTime=1/100  BusOutputAsStruct=on
  Actuator : Subsystem  Tag=VisuJoint  mask(PreScan Sink Block: VisuJoint){UniqueID=1958, Translate_ObjectID3D=Citroen_C3_2.WheelL0, Rotate_ObjectID3D=Citroen_C3_2.WheelL0, TimeStep=1/100, DisplayName=[]}
      mask prompts: UniqueID "Parent Unique ID"; Translate_ObjectID3D "Translate Object Name"; Rotate_ObjectID3D "Rotate Object Name"; TimeStep "Simulation Step"; DisplayName "Display Name"
      mask help:
      | The VisuJoint block provides a way to adapt the location and orientation of a part of an object.
      |
      | For more information, please click Help.
      settings: DeleteFcn=PreScanBlockDeleteFcn;
      mask Help: eval('openHelp(223)')
      mask Display: image(imread('Joint.png'))
  wires:
  WheelL0_Citroen_C3_2/1 -> Actuator/1(Joint)

== system TSR_Scenario_001_cs/WheelL0_Citroen_C3_3 ==
  WheelL0_Citroen_C3_3 : Inport  Tag=inport/JointActuator  OutDataTypeStr=Bus: PRESCAN_POSE_DATA  SampleTime=1/100  BusOutputAsStruct=on
  Actuator : Subsystem  Tag=VisuJoint  mask(PreScan Sink Block: VisuJoint){UniqueID=1967, Translate_ObjectID3D=Citroen_C3_3.WheelL0, Rotate_ObjectID3D=Citroen_C3_3.WheelL0, TimeStep=1/100, DisplayName=[]}
      mask prompts: UniqueID "Parent Unique ID"; Translate_ObjectID3D "Translate Object Name"; Rotate_ObjectID3D "Rotate Object Name"; TimeStep "Simulation Step"; DisplayName "Display Name"
      mask help:
      | The VisuJoint block provides a way to adapt the location and orientation of a part of an object.
      |
      | For more information, please click Help.
      settings: DeleteFcn=PreScanBlockDeleteFcn;
      mask Help: eval('openHelp(223)')
      mask Display: image(imread('Joint.png'))
  wires:
  WheelL0_Citroen_C3_3/1 -> Actuator/1(Joint)

== system TSR_Scenario_001_cs/WheelL0_Citroen_C3_4 ==
  WheelL0_Citroen_C3_4 : Inport  Tag=inport/JointActuator  OutDataTypeStr=Bus: PRESCAN_POSE_DATA  SampleTime=1/100  BusOutputAsStruct=on
  Actuator : Subsystem  Tag=VisuJoint  mask(PreScan Sink Block: VisuJoint){UniqueID=2027, Translate_ObjectID3D=Citroen_C3_4.WheelL0, Rotate_ObjectID3D=Citroen_C3_4.WheelL0, TimeStep=1/100, DisplayName=[]}
      mask prompts: UniqueID "Parent Unique ID"; Translate_ObjectID3D "Translate Object Name"; Rotate_ObjectID3D "Rotate Object Name"; TimeStep "Simulation Step"; DisplayName "Display Name"
      mask help:
      | The VisuJoint block provides a way to adapt the location and orientation of a part of an object.
      |
      | For more information, please click Help.
      settings: DeleteFcn=PreScanBlockDeleteFcn;
      mask Help: eval('openHelp(223)')
      mask Display: image(imread('Joint.png'))
  wires:
  WheelL0_Citroen_C3_4/1 -> Actuator/1(Joint)
